simulink model "deOlaso_final_ej3_sim"  (R2021a)
settings: Solver=VariableStepAuto  StartTime=0.0  StopTime=30  RelTol=1e-3
values from neighbouring files (symbols this model uses):
  ue = -1    [deOlaso_final_ej3.m]
  x1e = 2    [deOlaso_final_ej3.m]
  x2e = 1    [deOlaso_final_ej3.m]
  x3e = 1    [deOlaso_final_ej3.m]
  x4e = 0    [deOlaso_final_ej3.m]
  x5e = 0    [deOlaso_final_ej3.m]
  x6e = 0    [deOlaso_final_ej3.m]
  ye = x2e    (= 1)    [deOlaso_final_ej3.m]
libraries: cstblocks x1
settings Model: Creator=deolassa  LastModifiedBy=deolassa

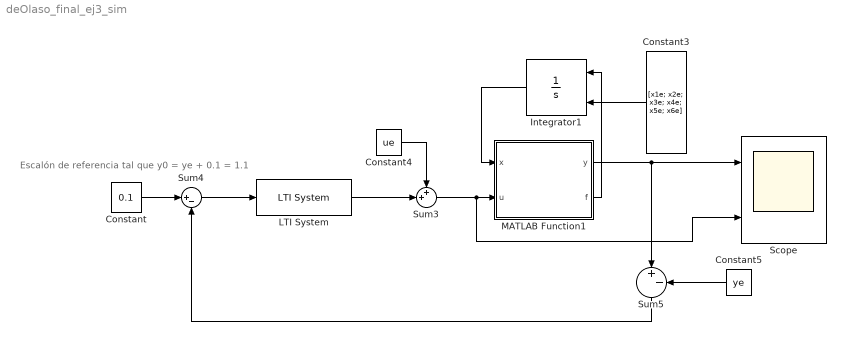
== system deOlaso_final_ej3_sim ==
  note: Escalón de referencia tal que y0 = ye + 0.1 = 1.1
  Constant : Constant  Value=0.1
  Constant3 : Constant  Value=[x1e; x2e; x3e; x4e; x5e; x6e]  VectorParams1D=off
  Constant4 : Constant  Value=ue
  Constant5 : Constant  Value=ye
  Integrator1 : Integrator  InitialConditionSource=external
  LTI System : cstblocks/LTI System  sys=C_digital  IC=[]
  MATLAB Function1 : MATLAB Function  TreatAsAtomicUnit=on
  Scope : Scope  NumInputPorts=2
  Sum3 : Sum  Inputs=++|
  Sum4 : Sum  Inputs=|+-
  Sum5 : Sum  Inputs=|+-
  wires:
  Constant4/1 -> Sum3/1
  Constant5/1 -> Sum5/2
  MATLAB Function1/1(y) -> Sum5/1, Scope/1
  LTI System/1 -> Sum3/2
  Integrator1/1 -> MATLAB Function1/1(x)
  Sum4/1 -> LTI System/1
  Constant3/1 -> Integrator1/2
  Sum5/1 -> Sum4/2
  MATLAB Function1/2(f) -> Integrator1/1
  Sum3/1 -> Scope/2, MATLAB Function1/2(u)
  Constant/1 -> Sum4/1

== matlab function deOlaso_final_ej3_sim/MATLAB Function1 ==
  data: x input; u input; y output; f output
function [y, f]= fcn(x, u)
    
p = 2;

f1 = (x(3) - sqrt(x(1) - x(2)))/(x(1)^2);
f2 = (sqrt(x(1)-x(2))) - sqrt(x(2))/(x(2)^2);
f3 = x(4);
f4 = x(5);
f5 = x(6);
f6 = -4*p*x(6) -6*(p^2)*x(5) -4*(p^3)*x(4) -(p^4)*x(3) + (p^4)*u;

% Lo que sale por la f son los x derivados
f = [f1; f2; f3; f4; f5; f6];

y = x(2);
